simulink model "stdp_synpase"  (Simulink 8.3)
settings: Solver=ode45  StartTime=0.0  StopTime=2  MaxStep=5e-4  RelTol=1e-3
values from neighbouring files (symbols this model uses):
  decay_n = 60    [test_stdp_synapse.m]
  decay_p = 200    [test_stdp_synapse.m]
  neg_gain = 0.7    [test_stdp_synapse.m]
  pos_gain = 0.7    [test_stdp_synapse.m]
  spike_period = [0.015]    [test_lif_neuron.m]    (also in test_stdp_synapse.m = (4 + 0.2*t_extra)/3*0.03)
  stdp_init_n = 20    [test_stdp_synapse.m]
  stdp_init_p = 20    [test_stdp_synapse.m]
  syn_decay = 0.01    [test_stdp_synapse.m]
  t_width = 0.05    [test_stdp_synapse.m]
libraries: simulink x3
settings Model: Creator=wjj  LastModifiedBy=wjj
settings DataIOCC: SignalLoggingSaveFormat=Dataset
settings DebuggingCC: UnderspecifiedInitializationDetection=Simplified  StateNameClashWarn=none
settings GRTTargetCC: CombineOutputUpdateFcns=on  GRTInterface=off

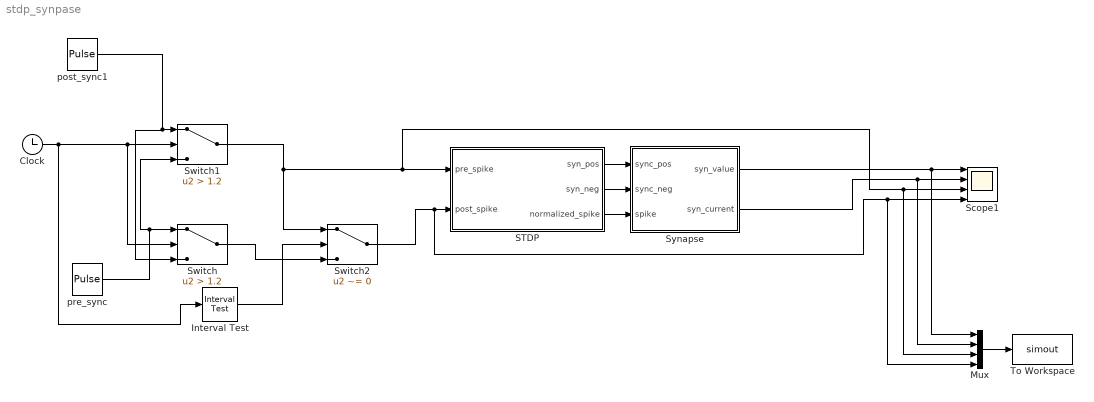
== system stdp_synpase ==
  Clock : Clock
  Interval Test : simulink/Logic and Bit Operations/Interval Test  IntervalClosedRight=on  uplimit=1.4  IntervalClosedLeft=on  lowlimit=1  OutDataTypeStr=boolean
  Mux : Mux
  STDP : Subsystem  mask{stdp_init_p=stdp_init_p, stdp_init_n=stdp_init_n, decay_p=decay_p, decay_n=decay_n, pos_gain=pos_gain, neg_gain=neg_gain}
      mask prompts: stdp_init_p "STDP positive initial value"; stdp_init_n "STDP negative initial value"; decay_p "Positive decay"; decay_n "Negative decay"; pos_gain "STDP positive gain"; neg_gain "STDP negative gain"
      mask DialogControl DescTextVar Prompt: STDP module receives pre-spikes and post spikes.
  Scope1 : Scope  NumInputPorts=4
      settings: TimeRange=0.2036836907593218  YMin=0~0~0~-5  YMax=12.5~15~0.175~5  SaveName=ScopeData10
  Switch : Switch  Criteria=u2 > Threshold  Threshold=1.2
  Switch1 : Switch  Criteria=u2 > Threshold  Threshold=1.2
  Switch2 : Switch  Criteria=u2 ~= 0  Threshold=1.2
  Synapse : Subsystem  mask{syn_decay=syn_decay}
      mask prompts: syn_decay "Synapse weigh decay"
      mask DialogControl DescTextVar Prompt: Synapse module receives delta weighs, and generates synapse current.
  To Workspace : ToWorkspace  VariableName=simout  SampleTime=5e-4
      settings: Save2DSignal=2-D array (concatenate along first dimension)
  post_sync1 : DiscretePulseGenerator  PulseType=Time based  Period=spike_period(1)  PulseWidth=t_width*100  PhaseDelay=5e-3
  pre_sync : DiscretePulseGenerator  PulseType=Time based  Period=spike_period(1)  PulseWidth=t_width*100
  wires:
  STDP/1(syn_pos) -> Synapse/1(sync_pos)
  STDP/2(syn_neg) -> Synapse/2(sync_neg)
  STDP/3(normalized_spike) -> Synapse/3(spike)
  Synapse/1(syn_value) -> Scope1/1, Mux/1
  Synapse/2(syn_current) -> Mux/2, Scope1/2
  Clock/1 -> Interval Test/1, Switch1/2, Switch/2
  pre_sync/1 -> Switch1/3, Switch/1
  post_sync1/1 -> Switch1/1, Switch/3
  Switch1/1 -> Switch2/1, Mux/3, Scope1/3, STDP/1(pre_spike)
  Switch2/1 -> Mux/4, Scope1/4, STDP/2(post_spike)
  Interval Test/1 -> Switch2/2
  Switch/1 -> Switch2/3
  Mux/1 -> To Workspace/1

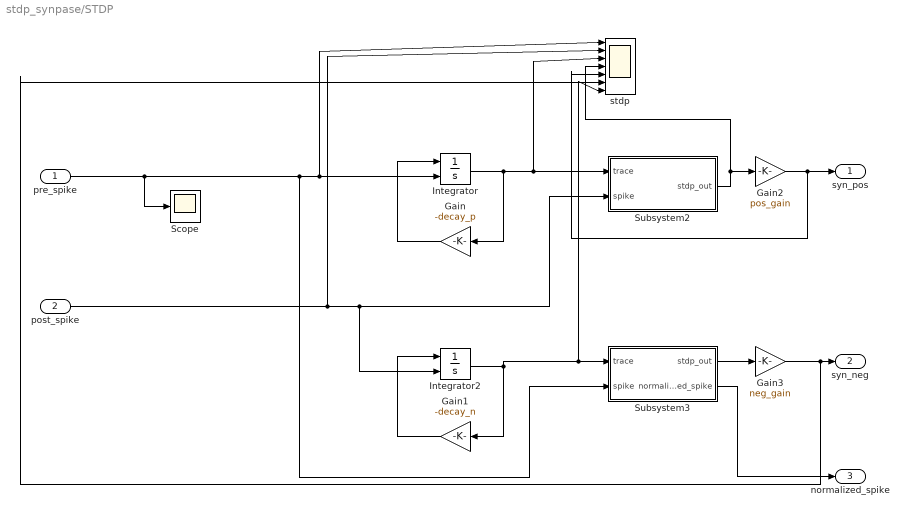
== system stdp_synpase/STDP ==
  pre_spike : Inport
  post_spike : Inport  Port=2
  Gain : Gain  Gain=-decay_p
  Gain1 : Gain  Gain=-decay_n
  Gain2 : Gain  Gain=pos_gain
  Gain3 : Gain  Gain=neg_gain
  Integrator : Integrator  ExternalReset=rising  InitialCondition=stdp_init_p  LowerSaturationLimit=0
  Integrator2 : Integrator  ExternalReset=rising  InitialCondition=stdp_init_n  LowerSaturationLimit=0
  Scope : Scope
      settings: SaveName=ScopeData6
  Subsystem2 : Subsystem
  Subsystem3 : Subsystem
  stdp : Scope  NumInputPorts=7
      settings: YMin=0~0~0~0~0~0~-5  YMax=1~1~20~20~15~15~5  SaveName=ScopeData5
  syn_pos : Outport
  syn_neg : Outport  Port=2
  normalized_spike : Outport  Port=3
  wires:
  post_spike/1 -> stdp/2, Subsystem2/2(spike), Integrator2/2
  pre_spike/1 -> Scope/1, Subsystem3/2(spike), stdp/1, Integrator/2
  Gain/1 -> Integrator/1
  Integrator2/1 -> Gain1/1, stdp/7, Subsystem3/1(trace)
  Subsystem3/1(stdp_out) -> Gain3/1
  Gain1/1 -> Integrator2/1
  Integrator/1 -> Subsystem2/1(trace), stdp/3, Gain/1
  Subsystem2/1(stdp_out) -> stdp/4, Gain2/1
  Gain3/1 -> stdp/6, syn_neg/1
  Subsystem3/2(normalized_spike) -> normalized_spike/1
  Gain2/1 -> stdp/5, syn_pos/1

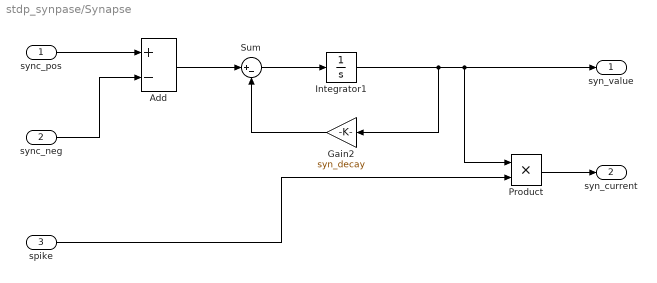
== system stdp_synpase/Synapse ==
  sync_pos : Inport
  sync_neg : Inport  Port=2
  spike : Inport  Port=3
  Add : Sum  Inputs=+-
  Gain2 : Gain  Gain=syn_decay
  Integrator1 : Integrator  InitialCondition=0.1  LimitOutput=on  UpperSaturationLimit=8  LowerSaturationLimit=0.1
  Product : Product
  Sum : Sum  Inputs=|+-
  syn_value : Outport
  syn_current : Outport  Port=2
  wires:
  sync_pos/1 -> Add/1
  sync_neg/1 -> Add/2
  Sum/1 -> Integrator1/1
  Integrator1/1 -> Gain2/1, syn_value/1, Product/1
  Gain2/1 -> Sum/2
  Add/1 -> Sum/1
  spike/1 -> Product/2
  Product/1 -> syn_current/1

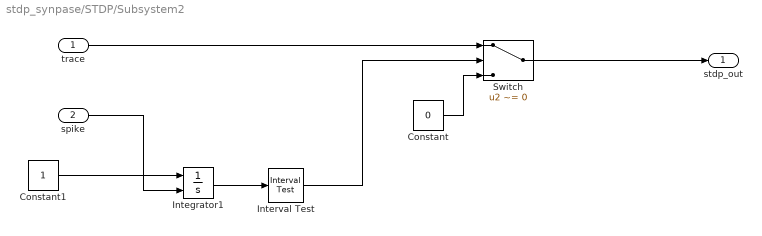
== system stdp_synpase/STDP/Subsystem2 ==
  trace : Inport
  spike : Inport  Port=2
  Constant : Constant  Value=0
  Constant1 : Constant
  Integrator1 : Integrator  ExternalReset=rising  LimitOutput=on  UpperSaturationLimit=2  LowerSaturationLimit=0
  Interval Test : simulink/Logic and Bit Operations/Interval Test  IntervalClosedRight=on  uplimit=1e-3  IntervalClosedLeft=on  lowlimit=0  OutDataTypeStr=boolean
  Switch : Switch  Criteria=u2 ~= 0  Threshold=0.05
  stdp_out : Outport
  wires:
  trace/1 -> Switch/1
  Constant/1 -> Switch/3
  Switch/1 -> stdp_out/1
  spike/1 -> Integrator1/2
  Constant1/1 -> Integrator1/1
  Integrator1/1 -> Interval Test/1
  Interval Test/1 -> Switch/2

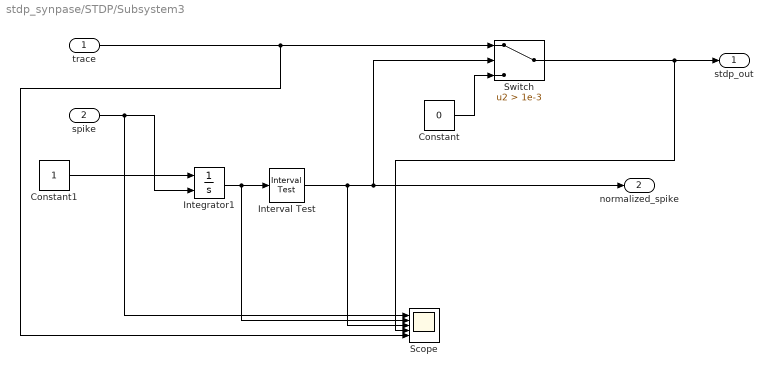
== system stdp_synpase/STDP/Subsystem3 ==
  trace : Inport
  spike : Inport  Port=2
  Constant : Constant  Value=0
  Constant1 : Constant
  Integrator1 : Integrator  ExternalReset=rising  LimitOutput=on  UpperSaturationLimit=2  LowerSaturationLimit=0
  Interval Test : simulink/Logic and Bit Operations/Interval Test  IntervalClosedRight=on  uplimit=1e-3  IntervalClosedLeft=on  lowlimit=0  OutDataTypeStr=boolean
  Scope : Scope  NumInputPorts=5
      settings: TimeRange=30  YMin=0~0~0~0~0  YMax=1~0.05~1~0.6~20  SaveName=ScopeData9
  Switch : Switch  Criteria=u2 > Threshold  Threshold=1e-3
  stdp_out : Outport
  normalized_spike : Outport  Port=2
  wires:
  trace/1 -> Scope/5, Switch/1
  Constant/1 -> Switch/3
  spike/1 -> Scope/1, Integrator1/2
  Constant1/1 -> Integrator1/1
  Integrator1/1 -> Interval Test/1, Scope/2
  Switch/1 -> Scope/4, stdp_out/1
  Interval Test/1 -> Scope/3, Switch/2, normalized_spike/1
